simulink model "antiwindup2"  (R2021a)
settings: Solver=VariableStepAuto  StartTime=0.0  StopTime=10.0  RelTol=1e-3
model workspace (MAT data in the model file):
  Kd = 0.01
  Ki = 1
  Kp = 0.8
  Threshold = 0.4
  umax = 0.6
  umin = -0.5
undefined symbols (not defined in the file): DiscIntNeverNeededParam
libraries: simulink x11
settings Model: Creator=治愈系的小木公子  LastModifiedBy=治愈系的小木公子

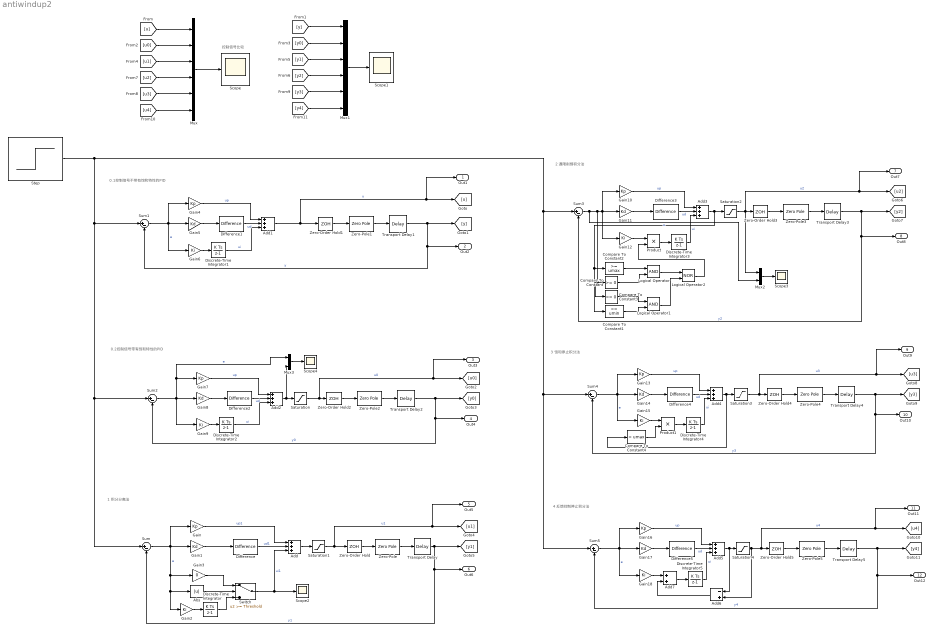
== system antiwindup2 ==
  note: 控制信号比较
  note: 1 积分分离法
  note: 0.1控制信号不带有饱和特性的PID
  note: 0.2控制信号带有饱和特性的PID
  note: 2 遇限削弱积分法
  note: 3 饱和停止积分法
  note: 4 反馈抑制停止积分法
  Abs : Abs
  Add{,1..5} (6 alike) : Sum  Inputs=+++
  Add6 : Sum  Inputs=-+
  Add7 : Sum
  Compare To Constant : simulink/Logic and Bit Operations/Compare To Constant  relop=>=  const=0  OutDataTypeStr=boolean
  Compare To Constant1 : simulink/Logic and Bit Operations/Compare To Constant  relop=<=  const=umin  OutDataTypeStr=boolean
  Compare To Constant2 : simulink/Logic and Bit Operations/Compare To Constant  relop=>=  const=umax  OutDataTypeStr=boolean
  Compare To Constant3 : simulink/Logic and Bit Operations/Compare To Constant  relop=<=  const=0  OutDataTypeStr=boolean
  Compare To Constant4 : simulink/Logic and Bit Operations/Compare To Constant  relop=<  const=umax  OutDataTypeStr=boolean
  Difference{,1..5} (6 alike) : simulink/Discrete/Difference  ICPrevInput=0.0  OutMin=[]  OutMax=[]  OutDataType=fixdt(1, 16)  OutScaling=2^-10  DoSatur=off
  Discrete-Time Integrator{,1..5} (6 alike) : DiscreteIntegrator  SampleTime=0.01  ICPrevOutput=DiscIntNeverNeededParam  ICPrevScaledInput=DiscIntNeverNeededParam
  Gain{,4,7,10,13,16} (6 alike) : Gain  Gain=Kp
  Gain{1,5,8,11,14,17} (6 alike) : Gain  Gain=Kd
  Gain{2,6,9,12,15,18} (6 alike) : Gain  Gain=Ki
  Gain3 : Gain  Gain=0
  Logical Operator : Logic  AllPortsSameDT=off  OutDataTypeStr=boolean
  Logical Operator1 : Logic  AllPortsSameDT=off  OutDataTypeStr=boolean
  Logical Operator2 : Logic  Operator=NOR  AllPortsSameDT=off  OutDataTypeStr=boolean
  Mux : Mux  Inputs=6
  Mux1 : Mux  Inputs=6
  Mux2 : Mux  Inputs=2
  Mux3 : Mux  Inputs=2
  Product : Product
  Product1 : Product
  Saturation{,1..4} (5 alike) : Saturate  UpperLimit=umax  LowerLimit=umin
  Scope{,1..4} (5 alike) : Scope
  Step : Step  SampleTime=0
  Sum{,1..5} (6 alike) : Sum  Inputs=|+-
  Switch : Switch  Threshold=Threshold
  Transport Delay{,1..5} (6 alike) : TransportDelay  DelayTime=0.1
  Zero-Order Hold{,1..5} (6 alike) : ZeroOrderHold  SampleTime=0.01
  Zero-Pole{,1..5} (6 alike) : ZeroPole  Zeros=[]  Poles=[0 -10]  Gain=10
  Out1 : Outport
  Out2 : Outport  Port=2
  Out3 : Outport  Port=3
  Out4 : Outport  Port=4
  Out5 : Outport  Port=5
  Out6 : Outport  Port=6
  Out7 : Outport  Port=7
  Out8 : Outport  Port=8
  Out9 : Outport  Port=9
  Out10 : Outport  Port=10
  Out11 : Outport  Port=11
  Out12 : Outport  Port=12
  wires:
  Sum/1 -> Abs/1, Gain2/1, Gain3/1, Gain/1, Gain1/1  "e"
  Gain2/1 -> Discrete-Time Integrator/1
  Abs/1 -> Switch/2
  Gain1/1 -> Difference/1
  Transport Delay/1 -> Sum/2, Out6/1, [y1]  "y1"
  Add/1 -> Saturation1/1
  Zero-Pole/1 -> Transport Delay/1
  Zero-Order Hold/1 -> Zero-Pole/1
  Gain/1 -> Add/1  "up1"
  Switch/1 -> Scope2/1, Add/3  "ui1"
  Difference/1 -> Add/2  "ud1"
  Difference1/1 -> Add1/2  "ud"
  Gain4/1 -> Add1/1  "up"
  Gain6/1 -> Discrete-Time Integrator1/1
  Transport Delay1/1 -> [y], Sum1/2, Out2/1  "y"
  Add1/1 -> Out1/1, [u], Zero-Order Hold1/1  "u"
  Sum1/1 -> Gain6/1, Gain4/1, Gain5/1  "e"
  Gain5/1 -> Difference1/1
  Zero-Pole1/1 -> Transport Delay1/1
  Zero-Order Hold1/1 -> Zero-Pole1/1
  Discrete-Time Integrator1/1 -> Add1/3  "ui"
  Gain9/1 -> Discrete-Time Integrator2/1
  Difference2/1 -> Add2/2  "ud"
  Gain7/1 -> Add2/1  "up"
  Transport Delay2/1 -> [y0], Sum2/2, Out4/1  "y0"
  Gain8/1 -> Difference2/1
  Sum2/1 -> Gain9/1, Mux3/1, Gain7/1, Gain8/1  "e"
  Zero-Pole2/1 -> Transport Delay2/1
  Discrete-Time Integrator2/1 -> Add2/3  "ui"
  Zero-Order Hold2/1 -> Zero-Pole2/1
  Saturation/1 -> Out3/1, [u0], Zero-Order Hold2/1  "u0"
  Add2/1 -> Mux3/2, Saturation/1
  Saturation1/1 -> Zero-Order Hold/1, Out5/1, [u1]  "u1"
  Mux/1 -> Scope/1
  [u] -> Mux/1
  [u0] -> Mux/2
  [u1] -> Mux/3
  Mux1/1 -> Scope1/1
  [y1] -> Mux1/3
  [y] -> Mux1/1
  [y0] -> Mux1/2
  Zero-Order Hold3/1 -> Zero-Pole3/1
  Transport Delay3/1 -> [y2], Out8/1, Sum3/2  "y2"
  Sum3/1 -> Mux2/2, Compare To Constant3/1, Compare To Constant/1, Gain12/1, Gain10/1, Gain11/1  "e"
  Saturation2/1 -> Mux2/1, Zero-Order Hold3/1, Out7/1, [u2]  "u2"
  Zero-Pole3/1 -> Transport Delay3/1
  Add3/1 -> Compare To Constant1/1, Compare To Constant2/1, Saturation2/1
  Gain11/1 -> Difference3/1
  Discrete-Time Integrator3/1 -> Add3/3  "ui"
  Gain10/1 -> Add3/1  "up"
  Difference3/1 -> Add3/2  "ud"
  Compare To Constant3/1 -> Logical Operator1/1
  Compare To Constant1/1 -> Logical Operator1/2
  Logical Operator/1 -> Logical Operator2/1
  Logical Operator1/1 -> Logical Operator2/2
  Compare To Constant/1 -> Logical Operator/2
  Compare To Constant2/1 -> Logical Operator/1
  [y2] -> Mux1/4
  [u2] -> Mux/4
  Gain12/1 -> Product/1
  Product/1 -> Discrete-Time Integrator3/1
  Logical Operator2/1 -> Product/2
  Step/1 -> Sum/1, Sum2/1, Sum1/1, Sum5/1, Sum4/1, Sum3/1
  Add4/1 -> Compare To Constant4/1, Saturation3/1
  Transport Delay4/1 -> [y3], Sum4/2, Out10/1  "y3"
  Discrete-Time Integrator4/1 -> Add4/3  "ui"
  Saturation3/1 -> Out9/1, [u3], Zero-Order Hold4/1  "u3"
  Zero-Order Hold4/1 -> Zero-Pole4/1
  Gain14/1 -> Difference4/1
  Difference4/1 -> Add4/2  "ud"
  Sum4/1 -> Gain15/1, Gain13/1, Gain14/1  "e"
  Zero-Pole4/1 -> Transport Delay4/1
  Gain13/1 -> Add4/1  "up"
  [y3] -> Mux1/5
  [u3] -> Mux/5
  Gain15/1 -> Product1/1
  Product1/1 -> Discrete-Time Integrator4/1
  Compare To Constant4/1 -> Product1/2
  Add7/1 -> Discrete-Time Integrator5/1
  Gain16/1 -> Add5/1  "up"
  Sum5/1 -> Gain18/1, Gain16/1, Gain17/1  "e"
  Zero-Pole5/1 -> Transport Delay5/1
  Difference5/1 -> Add5/2  "ud"
  Gain17/1 -> Difference5/1
  Zero-Order Hold5/1 -> Zero-Pole5/1
  Saturation4/1 -> Add6/2, Out11/1, [u4], Zero-Order Hold5/1  "u4"
  Discrete-Time Integrator5/1 -> Add5/3  "ui"
  Transport Delay5/1 -> [y4], Sum5/2, Out12/1  "y4"
  Add5/1 -> Add6/1, Saturation4/1
  [u4] -> Mux/6
  [y4] -> Mux1/6
  Gain18/1 -> Add7/1
  Add6/1 -> Add7/2
  Gain3/1 -> Switch/1
  Discrete-Time Integrator/1 -> Switch/3
  Mux2/1 -> Scope3/1
  Mux3/1 -> Scope4/1
